simulink model "sudarshan_simulink2"  (R2021b)
settings: Solver=VariableStepAuto  StartTime=0.0  StopTime=1000  RelTol=1e-3
libraries: simulink x1
settings Model: Creator=year2  LastModifiedBy=year2

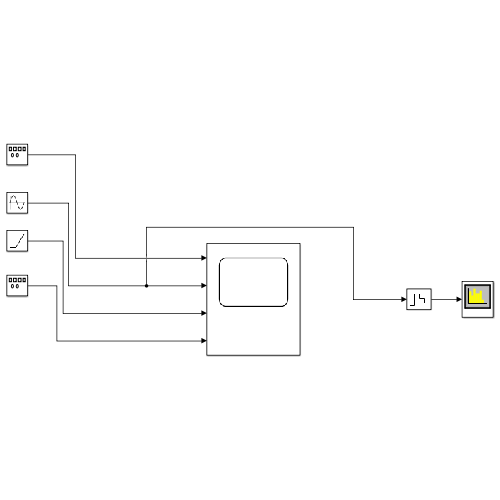
[thumbnail: Simulink's stored preview of the top-level diagram]
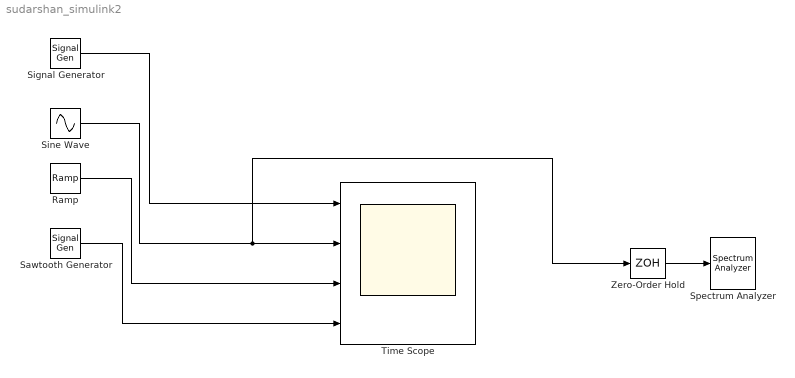
== system sudarshan_simulink2 ==
  Ramp : simulink/Sources/Ramp  slope=1  start=0  InitialOutput=0
  Sawtooth Generator : SignalGenerator  WaveForm=sawtooth  Units=rad/sec
  Signal Generator : SignalGenerator  Units=rad/sec
  Sine Wave : Sin  Frequency=100  SampleTime=0
  Spectrum Analyzer : SpectrumAnalyzer
  Time Scope : Scope  NumInputPorts=4
  Zero-Order Hold : ZeroOrderHold  SampleTime=-1
  wires:
  Signal Generator/1 -> Time Scope/1
  Zero-Order Hold/1 -> Spectrum Analyzer/1
  Sine Wave/1 -> Zero-Order Hold/1, Time Scope/2
  Ramp/1 -> Time Scope/3
  Sawtooth Generator/1 -> Time Scope/4
